simulink model "slexMulticoreExample"  (R2017b)
settings: Solver=FixedStepDiscrete  StartTime=0.0  StopTime=100  FixedStep=.1  RelTol=1e-3  EnableMultiTasking=on
Description:
  | Assign code to cores
settings Model: ParamWorkspaceSource=ReferencedWorkspace  ExtModeTrigMode=oneshot  ExtModeArmWhenConnect=off  ExtModeAutoUpdateStatusClock=off  ExplicitPartitioning=on  Creator=The MathWorks, Inc.  LastModifiedBy=The MathWorks, Inc.
settings SolverCC: ConcurrentTasks=on
settings DataIOCC: SaveFormat=StructureWithTime  SaveOutput=off  SaveTime=off  SignalLoggingName=sigsOut
settings OptimizationCC: BlockReduction=off  DefaultParameterBehavior=Inlined  UseDivisionForNetSlopeComputation=UseDivisionForReciprocalsOfIntegersOnly  InlineInvariantSignals=on  EnhancedBackFolding=on  ExpressionDepthLimit=2147483647  StateBitsets=on  DataBitsets=on  EfficientFloat2IntCast=on  LifeSpan=inf  BufferReusableBoundary=off
settings DebuggingCC: UnderspecifiedInitializationDetection=Classic  MergeDetectMultiDrivingBlocksExec=none  CheckExecutionContextPreStartOutputMsg=on  CheckExecutionContextRuntimeOutputMsg=on  IntegerOverflowMsg=none  FcnCallInpInsideContextMsg=warning  AllowSymbolicDim=off  StateNameClashWarn=warning  StrictBusMsg=ErrorOnBusTreatedAsVector  SFUnexpectedBacktrackingDiag=warning  SFNoUnconditionalDefaultTransitionDiag=warning  SFExecutionAtInitializationDiag=none  IntegerSaturationMsg=none
settings HardwareCC: ProdBitPerLong=64  ProdBitPerPointer=32  ProdBitPerSizeT=32  ProdBitPerPtrDiffT=32  ProdLargestAtomicFloat=None  ProdLongLongMode=on  ProdHWDeviceType=Specified  TargetHWDeviceType=Generic->32-bit Embedded Processor
settings ModelReferenceCC: UpdateModelReferenceTargets=IfOutOfDate  PropagateSignalLabelsOutOfModel=off
settings RTWCC: TLCOptions=-p0 -aWarnNonSaturatedBlocks=0  Description=Generic Real-Time Target  GenerateReport=on  RTWVerbose=off  RetainRTWFile=on  LaunchReport=on
settings CodeAppCC: ForceParamTrailComments=on  MaxIdLength=64  StateflowObjectComments=on
settings GRTTargetCC: TargetLangStandard=C89/C90 (ANSI)  UtilityFuncGeneration=Shared location  GeneratePreprocessorConditionals=Disable all  CombineOutputUpdateFcns=off  MatFileLogging=off  SupportNonFinite=off
settings ConfigComp: CovMetricSettings=d  CovHtmlReporting=on  CovSaveCumulativeToWorkspaceVar=on  CovSaveSingleToWorkspaceVar=on  CovExternalEMLEnable=off  CovSFcnEnable=off

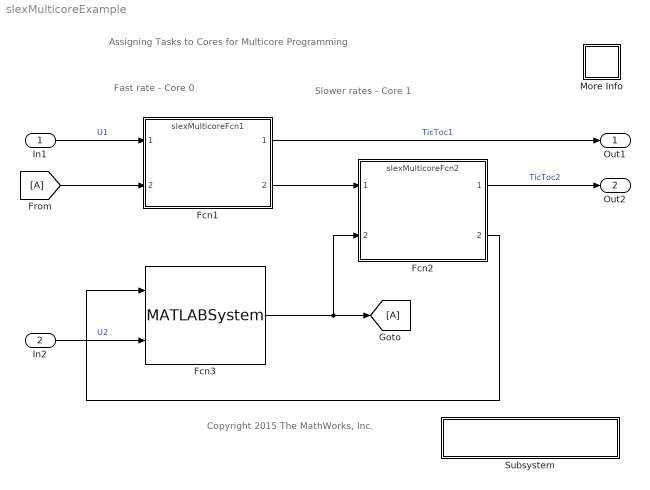
== system slexMulticoreExample ==
  note: Slower rates - Core 1
  note: Fast rate - Core 0
  note: Assigning Tasks to Cores for Multicore Programming
  note: Copyright 2015 The MathWorks, Inc.
  In1 : Inport  SampleTime=.1
  In2 : Inport  Port=2  OutDataTypeStr=double  PortDimensions=1
  Fcn1 : ModelReference  ModelNameDialog=slexMulticoreFcn1  SimulationMode=Normal  ModelReferenceVersion=1.262
  Fcn2 : ModelReference  ModelNameDialog=slexMulticoreFcn2  SimulationMode=Normal  ModelReferenceVersion=1.269
  Fcn3 : MATLABSystem  System=slexMulticoreFcn3  nIter=nIter  SimulateUsing=Interpreted execution
      mask Type: slexMulticoreFcn3
      mask Display:
      | disp('Fcn3');
      | port_label('input',1,'u1');
      | port_label('input',2,'u2');
      | port_label('output',1,'Multiplier');
  More Info : Subsystem
      settings: OpenFcn=showdemo('slexMulticoreExampleScript')
      mask Display: disp('?')
  Subsystem : Subsystem
      settings: OpenFcn=Simulink.architecture.profile(bdroot,20);
      mask Display: disp(sprintf('Generate Code and Profile Report\n(Double-Click)'));
  Out1 : Outport
  Out2 : Outport  Port=2
  wires:
  Fcn1/2 -> Fcn2/1
  Fcn2/2 -> Fcn3/1
  In1/1 -> Fcn1/1  "U1"
  In2/1 -> Fcn3/2  "U2"
  Fcn1/1 -> Out1/1  "TicToc1"
  Fcn2/1 -> Out2/1  "TicToc2"
  Fcn3/1 -> Fcn2/2, [A]
  [A] -> Fcn1/2

== system slexMulticoreExample/More Info ==

== system slexMulticoreExample/Subsystem ==
